simulink model "orbit_R2019b"  (R2019b)
settings: Solver=ode5  StartTime=0.0  StopTime=3600  FixedStep=1  RelTol=1e-3
values from neighbouring files (symbols this model uses):
  r0_I = A_FI*rF    [main.m]
  rEarth = 6.378137e6    (= 6378137)    [main.m]
  v0_I = A_FI*vF    [main.m]
undefined symbols (not defined in the file or in its folder): IAU
libraries: aerolibtransform2 x3, aerolibconvert2 x1, aerolibgravity2 x1
settings Model: Creator=tjones  LastModifiedBy=tjones

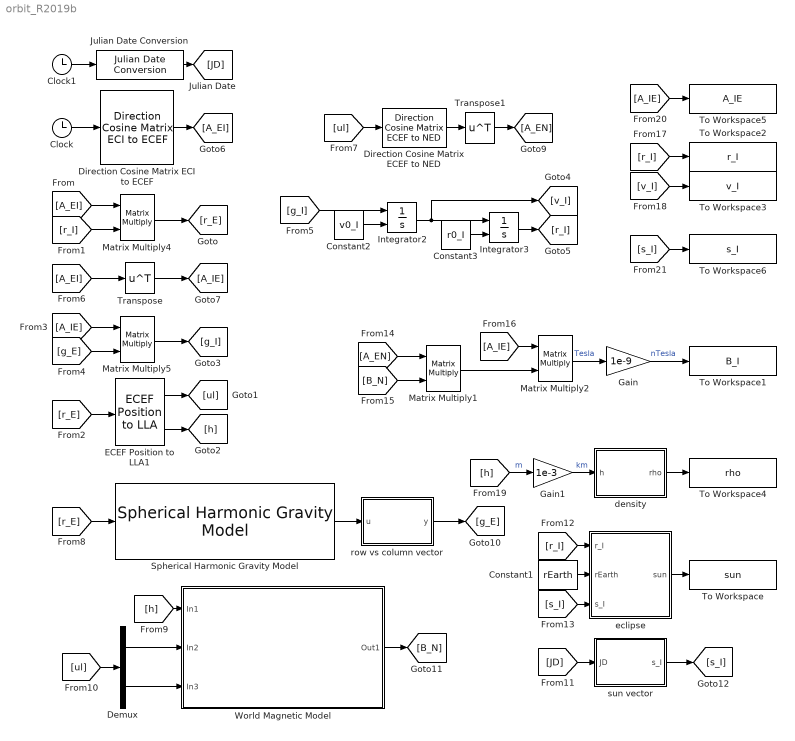
== system orbit_R2019b ==
  Clock : Clock
  Clock1 : Clock
  Constant1 : Constant  Value=rEarth
  Constant2 : Constant  Value=v0_I
  Constant3 : Constant  Value=r0_I
  Demux : Demux  Outputs=2
  Direction Cosine Matrix ECEF to NED : aerolibtransform2/Direction Cosine Matrix ECEF to NED
      settings: SourceProductBaseCode=AE
  Direction Cosine Matrix ECI to ECEF : aerolibtransform2/Direction Cosine Matrix ECI to ECEF  red=IAU-2000/2006  year=2021  month=March  day=1  hour=0  min=0  sec=0  deltaT=Sec  errorflag=Error  extraparamflag=off
      settings: AttributesFormatString=%<red>  SourceProductBaseCode=AE
  ECEF Position to LLA1 : aerolibtransform2/ECEF Position to LLA  R=6378137
  Gain : Gain  Gain=1e-9
  Gain1 : Gain  Gain=1e-3
  Integrator2 : Integrator  InitialConditionSource=external
  Integrator3 : Integrator  InitialConditionSource=external
  Julian Date Conversion : aerolibconvert2/Julian Date Conversion  year=2021  month=March  day=1  hour=0  min=0  sec=0  modflag=off  deltaT=Sec  errorflag=Error
      settings: SourceProductBaseCode=AE
  Matrix Multiply{1..2,4..5} (4 alike) : Product  Multiplication=Matrix(*)
  Spherical Harmonic Gravity Model : aerolibgravity2/Spherical Harmonic Gravity Model  units=Metric (MKS)  degree=21  action=Warning  ptype=EGM2008  datafile='aerogmm2b.mat'
      settings: SourceProductBaseCode=AE
  To Workspace : ToWorkspace  VariableName=sun  SaveFormat=Timeseries  SampleTime=-1
  To Workspace1 : ToWorkspace  VariableName=B_I  SaveFormat=Timeseries  SampleTime=-1
  To Workspace2 : ToWorkspace  VariableName=r_I  SaveFormat=Timeseries  SampleTime=-1
  To Workspace3 : ToWorkspace  VariableName=v_I  SaveFormat=Timeseries  SampleTime=-1
  To Workspace4 : ToWorkspace  VariableName=rho  SaveFormat=Timeseries  SampleTime=-1
  To Workspace5 : ToWorkspace  VariableName=A_IE  SaveFormat=Timeseries  SampleTime=-1
  To Workspace6 : ToWorkspace  VariableName=s_I  SaveFormat=Timeseries  SampleTime=-1
  Transpose : Math  Operator=transpose  SaturateOnIntegerOverflow=on
  Transpose1 : Math  Operator=transpose  SaturateOnIntegerOverflow=on
  World Magnetic Model : Subsystem  Description=Replaced Block  mask(Replaced Block){}
      mask help: This block has been replaced with an empty subsystem because it used functionality that is unavailable in Simulink R2019b.
      mask Display: fprintf('Replaced: %s\n','World Magnetic Model')
  density : MATLAB Function  TreatAsAtomicUnit=on
  eclipse : MATLAB Function  TreatAsAtomicUnit=on
  row vs column vector : MATLAB Function  TreatAsAtomicUnit=on
  sun vector : MATLAB Function  TreatAsAtomicUnit=on
  wires:
  Clock/1 -> Direction Cosine Matrix ECI to ECEF/1
  Demux/1 -> World Magnetic Model/2(In2)
  Demux/2 -> World Magnetic Model/3(In3)
  Direction Cosine Matrix ECEF to NED/1 -> Transpose1/1
  Clock1/1 -> Julian Date Conversion/1
  Matrix Multiply4/1 -> [r_E]
  [A_EI] -> Matrix Multiply4/1
  [r_I] -> Matrix Multiply4/2
  [r_E] -> ECEF Position to LLA1/1
  ECEF Position to LLA1/1 -> [ul]
  ECEF Position to LLA1/2 -> [h]
  [g_E] -> Matrix Multiply5/2
  [A_IE] -> Matrix Multiply5/1
  Matrix Multiply5/1 -> [g_I]
  Integrator2/1 -> [v_I], Integrator3/1
  Constant3/1 -> Integrator3/2
  Constant2/1 -> Integrator2/2
  [g_I] -> Integrator2/1
  Integrator3/1 -> [r_I]
  Direction Cosine Matrix ECI to ECEF/1 -> [A_EI]
  [A_EI] -> Transpose/1
  Transpose/1 -> [A_IE]
  Julian Date Conversion/1 -> [JD]
  [ul] -> Direction Cosine Matrix ECEF to NED/1
  Transpose1/1 -> [A_EN]
  [r_E] -> Spherical Harmonic Gravity Model/1
  [h] -> World Magnetic Model/1(In1)
  [ul] -> Demux/1
  World Magnetic Model/1(Out1) -> [B_N]
  [JD] -> sun vector/1(JD)
  sun vector/1(s_I) -> [s_I]
  [r_I] -> eclipse/1(r_I)
  Constant1/1 -> eclipse/2(rEarth)
  [s_I] -> eclipse/3(s_I)
  eclipse/1(sun) -> To Workspace/1
  [B_N] -> Matrix Multiply1/2
  [A_EN] -> Matrix Multiply1/1
  [A_IE] -> Matrix Multiply2/1
  Matrix Multiply1/1 -> Matrix Multiply2/2
  Matrix Multiply2/1 -> Gain/1  "Tesla"
  Gain/1 -> To Workspace1/1  "nTesla"
  [r_I] -> To Workspace2/1
  [v_I] -> To Workspace3/1
  density/1(rho) -> To Workspace4/1
  [A_IE] -> To Workspace5/1
  [s_I] -> To Workspace6/1
  [h] -> Gain1/1  "m"
  Gain1/1 -> density/1(h)  "km"
  row vs column vector/1(y) -> [g_E]
  Spherical Harmonic Gravity Model/1 -> row vs column vector/1(u)

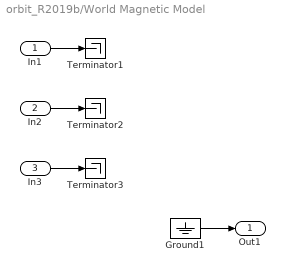
== system orbit_R2019b/World Magnetic Model ==
  In1 : Inport
  In2 : Inport  Port=2
  In3 : Inport  Port=3
  Ground1 : Ground
  Terminator1 : Terminator
  Terminator2 : Terminator
  Terminator3 : Terminator
  Out1 : Outport
  wires:
  Ground1/1 -> Out1/1
  In3/1 -> Terminator3/1
  In2/1 -> Terminator2/1
  In1/1 -> Terminator1/1

== matlab function orbit_R2019b/row vs column vector ==
  data: u input; y output
function y = fcn(u)

y = u';

== matlab function orbit_R2019b/sun vector ==
  data: JD input; s_I output
function s_I = fcn(JD)

s_I = get_sunvector(JD);

== matlab function orbit_R2019b/eclipse ==
  data: r_I input; sun output; rEarth input; s_I input
function sun = fcn(r_I, rEarth, s_I)

sun = 1;
if get_eclipse(r_I, rEarth, s_I)
    sun = 0;
end

== matlab function orbit_R2019b/density ==
  data: h input; rho output
function rho = fcn(h)
rho = get_density(h);
